simulink model "SFF_Simulator"  (R2024a)
settings: Solver=FixedStepAuto  StartTime=0.0  StopTime=tf  FixedStep=step_modelo  RelTol=1e-3
values from neighbouring files (symbols this model uses):
  AttKd_x = inp(4,2).Var2    [SFF_Simulator_Entradas.m]
  AttKd_y = inp(5,2).Var2    [SFF_Simulator_Entradas.m]
  AttKd_z = inp(6,2).Var2    [SFF_Simulator_Entradas.m]
  AttKp_x = inp(1,2).Var2    [SFF_Simulator_Entradas.m]
  AttKp_y = inp(2,2).Var2    [SFF_Simulator_Entradas.m]
  AttKp_z = inp(3,2).Var2    [SFF_Simulator_Entradas.m]
  beta = inp(2,2).Var2    [SFF_Simulator_Entradas.m]
  cdgps = inp(1,2).Var2    [SFF_Simulator_Entradas.m]
  estrelas = inp(4,2).Var2    [SFF_Simulator_Entradas.m]
  estrelas_bias = inp(6,2).Var2    [SFF_Simulator_Entradas.m]
  estrelas_ruido = inp(5,2).Var2    [SFF_Simulator_Entradas.m]
  gps_bias = inp(3,2).Var2    [SFF_Simulator_Entradas.m]
  gps_ruido = inp(2,2).Var2    [SFF_Simulator_Entradas.m]
  m1 = inp(6,2).Var2    [SFF_Simulator_Entradas.m]
  magne = inp(10,2).Var2    [SFF_Simulator_Entradas.m]
  magne_bias = inp(12,2).Var2    [SFF_Simulator_Entradas.m]
  magne_ruido = inp(11,2).Var2    [SFF_Simulator_Entradas.m]
  man = inp(1,2).Var2    [SFF_Simulator_Entradas.m]
  OrbKd_x = inp(3,2).Var2    [SFF_Simulator_Entradas.m]
  OrbKd_y = inp(6,2).Var2    [SFF_Simulator_Entradas.m]
  OrbKd_z = inp(9,2).Var2    [SFF_Simulator_Entradas.m]
  OrbKi_x = inp(2,2).Var2    [SFF_Simulator_Entradas.m]
  OrbKi_y = inp(5,2).Var2    [SFF_Simulator_Entradas.m]
  OrbKi_z = inp(8,2).Var2    [SFF_Simulator_Entradas.m]
  OrbKp_x = inp(1,2).Var2    [SFF_Simulator_Entradas.m]
  OrbKp_y = inp(4,2).Var2    [SFF_Simulator_Entradas.m]
  OrbKp_z = inp(7,2).Var2    [SFF_Simulator_Entradas.m]
  propForcaAtivo = inp(1,2).Var2    [SFF_Simulator_Entradas.m]
  rodaAtivo = inp(1,2).Var2    [SFF_Simulator_Entradas.m]
  torqrodAtivo = inp(1,2).Var2    [SFF_Simulator_Entradas.m]
undefined symbols (not defined in the file or in its folder): IAU, WMM2020
libraries: dspsrcs4 x9, aerolibtransform2 x1, aerolibgravity2 x1
(part 2 of 2)

== matlab function SFF_Simulator/Erros Quatérnions/MATLAB Function4 ==
  data: q_d input; q_error output; q input
function q_error = fcn(q_d,q)

qt1 = q_d(1);
qt2 = q_d(2);
qt3 = q_d(3);
qt4 = q_d(4);

qs1 = q(1);
qs2 = q(2);
qs3 = q(3);
qs4 = q(4);

q_error = [qt4 qt3 -qt2 qt1
    -qt3 qt4 qt1 qt2
    qt2 -qt1 qt4 qt3
    -qt1 -qt2 -qt3 qt4]*[-qs1;-qs2;-qs3;qs4];

== matlab function SFF_Simulator/Guiamento Atitude/Euler -> Quatérnions ==
  data: phi_ref input; q_ref output; theta_ref input; psi_ref input
function q_ref = fcn(phi_ref,theta_ref,psi_ref)

q_ref = eul2quat([phi_ref theta_ref psi_ref]);

q_ref = [q_ref(2),q_ref(3),q_ref(4),q_ref(1)];

== matlab function SFF_Simulator/Sensores Atitude/Euler -> Quat ==
  data: phi_ref input; q_ref output; theta_ref input; psi_ref input; q_in input
function q_ref = fcn(phi_ref,theta_ref,psi_ref,q_in)

q_ref = eul2quat([phi_ref theta_ref psi_ref]);

q_ref = [sign(q_in(1))*abs(q_ref(2)),sign(q_in(2))*abs(q_ref(3)),sign(q_in(3))*abs(q_ref(4)),sign(q_in(4))*abs(q_ref(1))];

== matlab function SFF_Simulator/Sensores Atitude/Quat -> Euler ==
  data: u input; phi output; theta output; psi output
function [phi,theta,psi] = fcn(u)

y = quat2eul([u(4) u(1) u(2) u(3)]);

phi = (y(1)); 
theta = (y(2));
psi = (y(3));
